simulink model "Model_1_PI_Gain_Test"  (R2017b)
settings: Solver=VariableStepAuto  StartTime=0.0  StopTime=1  MaxStep=1e-5  RelTol=1e-3  EnableMultiTasking=on
values from neighbouring files (symbols this model uses):
  Gain_I = 1    [Model_1_init.m]    (also in Model_2_init.m = 26.84; Model_3_init.m = 26.84)
  Gain_P = 1    [Model_1_init.m]    (also in Model_2_init.m = 7.74; Model_3_init.m = 7.74)
  Id_reference = -50    [Model_1_init.m]
  Iq_reference = 100    [Model_1_init.m]
  Lambda_m = 0.2205    [Model_1_init.m]    (also in Model_2_init.m; Model_3_init.m)
  Ld = 1.7e-3    (= 0.0017)    [Model_1_init.m]    (also in Model_2_init.m; Model_3_init.m)
  Lq = 3.2e-3    (= 0.0032)    [Model_1_init.m]    (also in Model_2_init.m; Model_3_init.m)
  Polepairs = 4    [Model_1_init.m]    (also in Model_2_init.m; Model_3_init.m)
  Rs = 0.02    [Model_1_init.m]    (also in Model_2_init.m; Model_3_init.m)
libraries: powerlib x19, simulink x5, powerlib_meascontrol x1
settings Model: SimulationMode=accelerator  Creator=dakaihu  LastModifiedBy=proso
settings DataIOCC: LimitDataPoints=on
settings OptimizationCC: LifeSpan=inf
settings DebuggingCC: AllowSymbolicDim=off  SFUnexpectedBacktrackingDiag=warning  SFNoUnconditionalDefaultTransitionDiag=warning  SFExecutionAtInitializationDiag=none
settings ModelReferenceCC: PropagateSignalLabelsOutOfModel=off
settings CodeAppCC: StateflowObjectComments=on
settings GRTTargetCC: TargetLangStandard=C89/C90 (ANSI)
settings ConfigComp: CovMetricSettings=dw  CovSaveCumulativeToWorkspaceVar=on  CovSaveSingleToWorkspaceVar=on  CovExternalEMLEnable=off
settings SimscapeCC: SimscapeNormalizeSystem=off

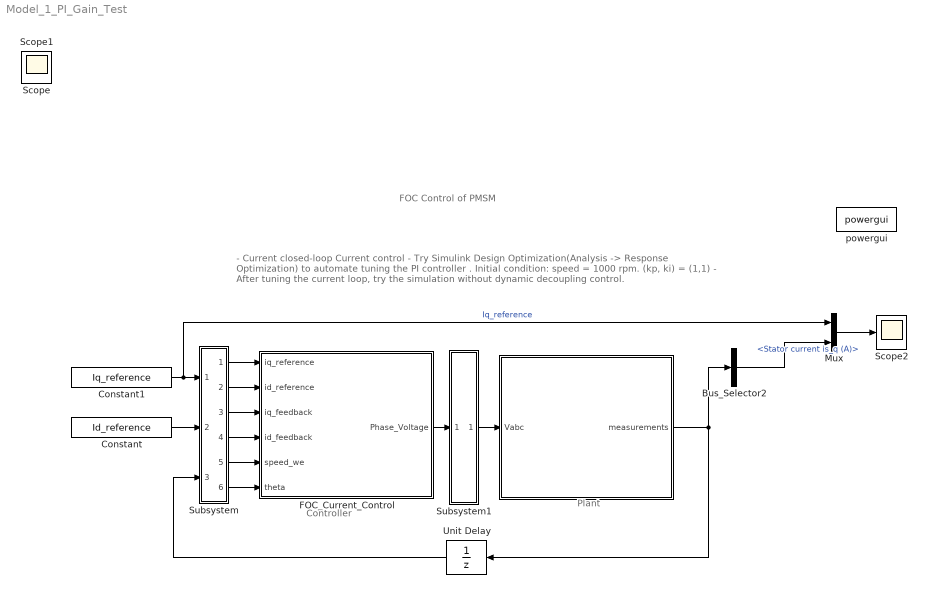
== system Model_1_PI_Gain_Test ==
  note: - Current closed-loop Current control
      | - Try Simulink Design Optimization(Analysis -> Response Optimization) to automate tuning the PI controller .  Initial condition: speed = 1000 rpm. (kp, ki) = (1,1)
      | - After tuning the current loop, try the simulation without dynamic decoupling control.
  note: Controller
  note: Plant
  note: FOC Control of PMSM
  " " : Subsystem
  Bus_Selector2 : BusSelector  OutputSignals=Stator current is_q (A)
  Constant : Constant  Value=Id_reference
  Constant1 : Constant  Value=Iq_reference  VectorParams1D=off
  FOC_Current_Control : Subsystem
  Mux : Mux  Inputs=2
  Scope2 : Scope
  Subsystem : Subsystem
      mask Display: fprintf('C/D')
  Subsystem1 : Subsystem
      mask Display: fprintf('D/C')
  Unit Delay : UnitDelay  SampleTime=1e-4
  powergui : powerlib/powergui  SimulationMode=Continuous  SampleTime=1e-5  frequency=60  Iterations=50  frequencyindice=0  Pbase=100e6  ErrMax=1e-4  UnitsV=kV  UnitsW=MW  buscounter=0  FunctionMessages=off  echomessages=off  EnableUseOfTLC=off  CurrentSourceSwitches=off  DisableSnubberDevices=off  DisableRonSwitches=off  DisableVfSwitches=off  DisplayEquations=off  SolverType=Tustin/Backward Euler (TBE)  Interpol=off  ExternalGateDelay=off  methode=off  Ts=100  x0status=blocks  SPID=on  SwTol=0  HookPort=off  RestoreLinks=warning  ResistiveCurrentMeasurement=off  Frange=[0:2:500]  Ylog=off  Xlog=on  ShowGrid=off  save=off  variable=ZData  structure=0  ZoomFFT=on  StartTime=0.0  cycles=1  DisplayStyle=1  fundamental=60  FreqAxis=off  MaxFrequency=1000  frequencyindicesteady=1  RmsSteady=1  display=off
  Scope : Scope
  Scope1 : Scope
  wires:
  FOC_Current_Control/1(Phase_Voltage) -> Subsystem1/1(In1)
  " "/1(measurements) -> Unit Delay/1, Bus_Selector2/1
  Subsystem/3(Out2) -> FOC_Current_Control/3(iq_feedback)
  Subsystem/4(Out3) -> FOC_Current_Control/4(id_feedback)
  Subsystem1/1(Out1) -> " "/1(Vabc)
  Unit Delay/1 -> Subsystem/3(PMSM_Measurements)
  Subsystem/5(Out1) -> FOC_Current_Control/5(speed_we)
  Subsystem/6(Out4) -> FOC_Current_Control/6(theta)
  Mux/1 -> Scope2/1
  Bus_Selector2/1 -> Mux/2  "<Stator current is_q (A)>"
  Constant/1 -> Subsystem/2(id_ref)
  Constant1/1 -> Mux/1, Subsystem/1(iq_ref)  "Iq_reference"
  Subsystem/1(Out6) -> FOC_Current_Control/1(iq_reference)
  Subsystem/2(Out5) -> FOC_Current_Control/2(id_reference)

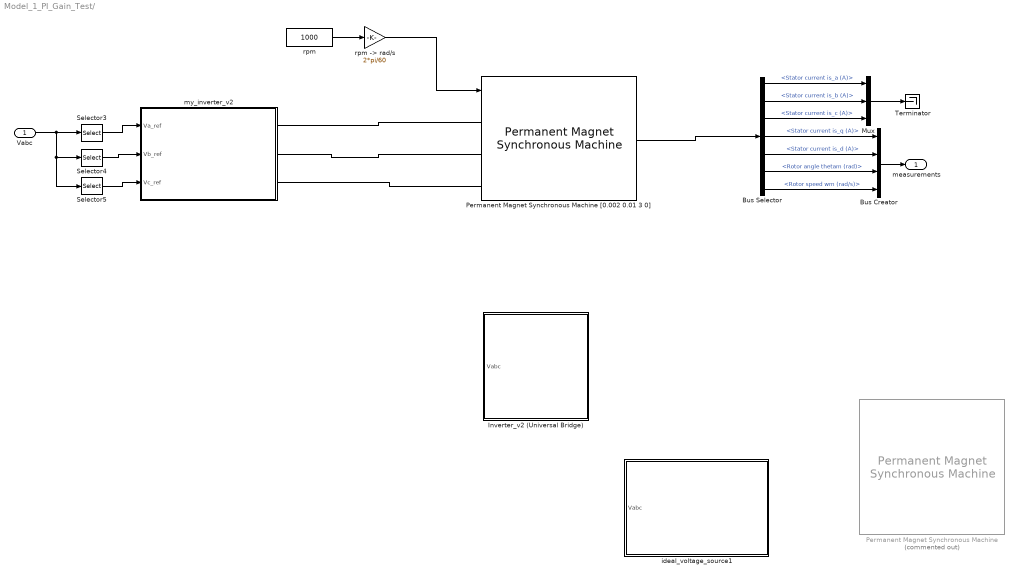
== system Model_1_PI_Gain_Test/  ==
  Vabc : Inport
  " Inverter_v2 (Universal Bridge)" : Subsystem
  Bus Creator : BusCreator  Inputs=4
  Bus Selector : BusSelector  OutputSignals=Stator current is_a (A),Stator current is_b (A),Stator current is_c (A),Stator current is_q (A),Stator current is_d (A),Rotor angle thetam (rad),Rotor speed wm (rad/s)
  Mux : Mux  Inputs=3
  Permanent Magnet Synchronous Machine : powerlib/Machines/Permanent Magnet Synchronous Machine  Commented=on  NbPhases=3  FluxDistribution=Sinusoidal  RotorType=Salient-pole  MechanicalLoad=Speed w  PresetModel=No  ShowDetailedParameters=on  MeasurementBus=off  Resistance=Rs  Inductance=8.5e-3  dqInductances=[Ld,Lq]  La=[Ld,Lq]  MachineConstant=Flux linkage established by magnets (V.s)  Flux=Lambda_m  VoltageCst=159.9771  TorqueCst=1.323  Flat=120  Mechanical=[0.0027 0.0004924 4 0]  PolePairs=Polepairs  InitialConditions=[0,0.01,3,0]  InitialConditions5ph=[0 0 0 0 0 0]  TsPowergui=0  TsBlock=-1  RefAngle=90 degrees behind phase A axis (modified Park)
      settings: SourceProductName=Simscape Power Systems
  Permanent Magnet Synchronous Machine [0.002 0.01 3 0] : powerlib/Machines/Permanent Magnet Synchronous Machine  NbPhases=3  FluxDistribution=Sinusoidal  RotorType=Salient-pole  MechanicalLoad=Speed w  PresetModel=No  ShowDetailedParameters=on  MeasurementBus=off  Resistance=Rs  Inductance=8.5e-3  dqInductances=[Ld,Lq]  La=0.000395  MachineConstant=Flux linkage established by magnets (V.s)  Flux=Lambda_m  VoltageCst=159.9771  TorqueCst=1.323  Flat=120  Mechanical=[0.0027 0.001 4 0]  PolePairs=Polepairs  InitialConditions=[0,0, 0,0]  InitialConditions5ph=[0 0 0 0 0 0]  TsPowergui=0  TsBlock=-1  RefAngle=Aligned with phase A axis (original Park)
  Selector3 : Selector  InputPortWidth=3  IndexOptions=Index vector (dialog)  Indices=[1]  OutputSizes=1
  Selector4 : Selector  InputPortWidth=3  IndexOptions=Index vector (dialog)  Indices=2  OutputSizes=1
  Selector5 : Selector  InputPortWidth=3  IndexOptions=Index vector (dialog)  Indices=3  OutputSizes=1
  Terminator : Terminator
  ideal_voltage_source1 : Subsystem  VariantControl=variantPwm == enumPwm.behavior
  my_inverter_v2 : Subsystem
  rpm : Constant  Value=1000
  "rpm -> rad/s" : Gain  Gain=2*pi/60
  measurements : Outport
  wires:
  rpm/1 -> "rpm -> rad/s"/1
  Bus Selector/4 -> Bus Creator/1  "<Stator current is_q (A)>"
  Bus Selector/5 -> Bus Creator/2  "<Stator current is_d (A)>"
  Bus Selector/6 -> Bus Creator/3  "<Rotor angle thetam (rad)>"
  Bus Creator/1 -> measurements/1
  Bus Selector/1 -> Mux/1  "<Stator current is_a (A)>"
  Bus Selector/2 -> Mux/2  "<Stator current is_b (A)>"
  Bus Selector/3 -> Mux/3  "<Stator current is_c (A)>"
  Mux/1 -> Terminator/1
  Permanent Magnet Synchronous Machine [0.002 0.01 3 0]/1 -> Bus Selector/1
  Bus Selector/7 -> Bus Creator/4  "<Rotor speed wm (rad/s)>"
  Vabc/1 -> Selector5/1, Selector4/1, Selector3/1
  Selector4/1 -> my_inverter_v2/2(Vb_ref)
  Selector3/1 -> my_inverter_v2/1(Va_ref)
  Selector5/1 -> my_inverter_v2/3(Vc_ref)
  "rpm -> rad/s"/1 -> Permanent Magnet Synchronous Machine [0.002 0.01 3 0]/1
  connections:
  my_inverter_v2/RConn1 -- Permanent Magnet Synchronous Machine [0.002 0.01 3 0]/LConn1
  my_inverter_v2/RConn2 -- Permanent Magnet Synchronous Machine [0.002 0.01 3 0]/LConn2
  my_inverter_v2/RConn3 -- Permanent Magnet Synchronous Machine [0.002 0.01 3 0]/LConn3

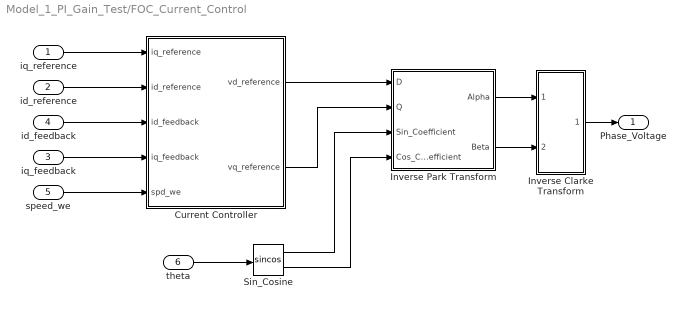
== system Model_1_PI_Gain_Test/FOC_Current_Control ==
  iq_reference : Inport  SampleTime=1e-4
  id_reference : Inport  Port=2  SampleTime=1e-4
  iq_feedback : Inport  Port=3  SampleTime=1e-4
  id_feedback : Inport  Port=4  SampleTime=1e-4
  speed_we : Inport  Port=5  SampleTime=1e-4
  theta : Inport  Port=6  SampleTime=1e-4
  Current Controller : Subsystem
  Inverse Clarke Transform : Subsystem
  Inverse Park Transform : Subsystem
  Sin_Cosine : Trigonometry  Operator=sincos
  Phase_Voltage : Outport  SampleTime=1e-4
  wires:
  Inverse Clarke Transform/1(ABC) -> Phase_Voltage/1
  Sin_Cosine/2 -> Inverse Park Transform/4(Cos_Coefficient)
  Sin_Cosine/1 -> Inverse Park Transform/3(Sin_Coefficient)
  theta/1 -> Sin_Cosine/1
  Current Controller/2(vq_reference) -> Inverse Park Transform/2(Q)
  Current Controller/1(vd_reference) -> Inverse Park Transform/1(D)
  Inverse Park Transform/1(Alpha) -> Inverse Clarke Transform/1(Alpha)
  Inverse Park Transform/2(Beta) -> Inverse Clarke Transform/2(Beta)
  id_feedback/1 -> Current Controller/3(id_feedback)
  iq_feedback/1 -> Current Controller/4(iq_feedback)
  speed_we/1 -> Current Controller/5(spd_we)
  iq_reference/1 -> Current Controller/1(iq_reference)
  id_reference/1 -> Current Controller/2(id_reference)

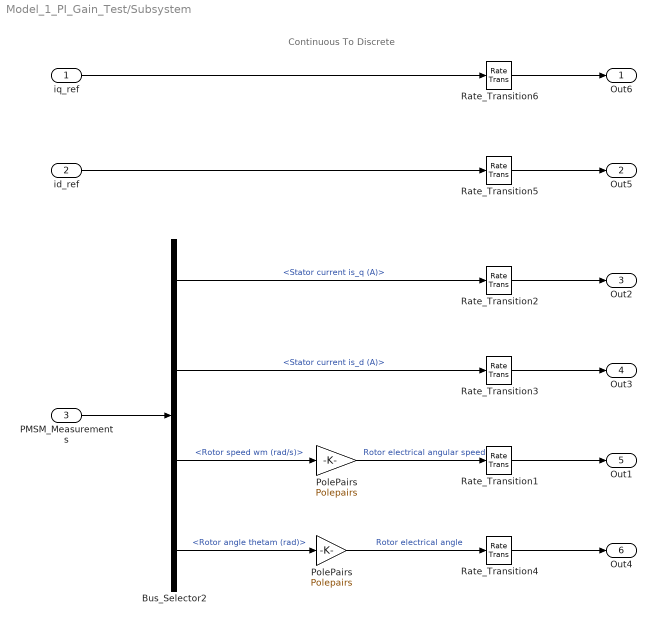
== system Model_1_PI_Gain_Test/Subsystem ==
  note: Continuous To Discrete
  iq_ref : Inport
  id_ref : Inport  Port=2
  PMSM_Measurements : Inport  Port=3
  Bus_Selector2 : BusSelector  OutputSignals=Stator current is_q (A),Stator current is_d (A),Rotor speed wm (rad/s),Rotor angle thetam (rad)
  PolePairs : Gain  Gain=Polepairs
  "PolePairs " : Gain  Gain=Polepairs
  Rate_Transition{1..6} (6 alike) : RateTransition  Integrity=off  Deterministic=off
  Out6 : Outport
  Out5 : Outport  Port=2
  Out2 : Outport  Port=3
  Out3 : Outport  Port=4
  Out1 : Outport  Port=5
  Out4 : Outport  Port=6
  wires:
  Rate_Transition4/1 -> Out4/1
  Bus_Selector2/2 -> Rate_Transition3/1  "<Stator current is_d (A)>"
  id_ref/1 -> Rate_Transition5/1
  iq_ref/1 -> Rate_Transition6/1
  Bus_Selector2/1 -> Rate_Transition2/1  "<Stator current is_q (A)>"
  Bus_Selector2/4 -> PolePairs/1  "<Rotor angle thetam (rad)>"
  PMSM_Measurements/1 -> Bus_Selector2/1
  PolePairs/1 -> Rate_Transition4/1  "Rotor electrical angle"
  Rate_Transition5/1 -> Out5/1
  Rate_Transition6/1 -> Out6/1
  Rate_Transition2/1 -> Out2/1
  Rate_Transition3/1 -> Out3/1
  Rate_Transition1/1 -> Out1/1
  Bus_Selector2/3 -> "PolePairs "/1  "<Rotor speed wm (rad/s)>"
  "PolePairs "/1 -> Rate_Transition1/1  "Rotor electrical angular speed"

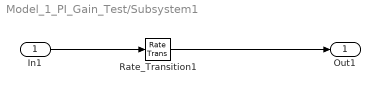
== system Model_1_PI_Gain_Test/Subsystem1 ==
  In1 : Inport
  Rate_Transition1 : RateTransition  Integrity=off
  Out1 : Outport
  wires:
  In1/1 -> Rate_Transition1/1
  Rate_Transition1/1 -> Out1/1

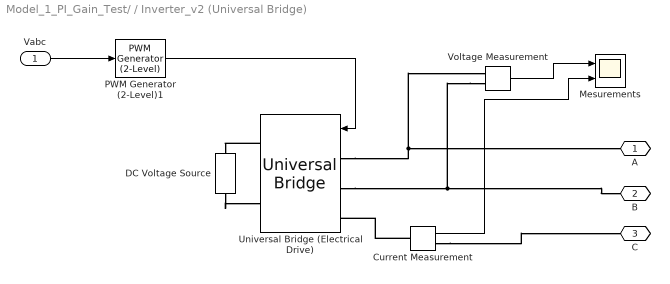
== system Model_1_PI_Gain_Test/ / Inverter_v2 (Universal Bridge) ==
  Vabc : Inport
  Current Measurement : powerlib/Measurements/Current Measurement  PhasorSimulation=off  OutputType=Complex  PSBequivalent=0
  DC Voltage Source : powerlib/Electrical Sources/DC Voltage Source  Amplitude=100  Measurements=None
  Mesurements : Scope  NumInputPorts=2
  PWM Generator (2-Level)1 : powerlib_meascontrol/Pulse & Signal Generators/PWM Generator (2-Level)  ModulatorType=Three-phase bridge (6 pulses)  ModulatorMode=Unsynchronized  Fc=27*60  Pc=90  nF=27  MinMax="[ -1  1 ]"  SamplingTechnique=Natural  ModulatingSignals=off  m=0.8  Freq=60  Phase=0  Ts=0  ShowCarrierOutport=off
      settings: SourceProductName=Simscape Power Systems
  Universal Bridge (Electrical Drive) : powerlib/Power Electronics/Universal Bridge  Arms=3  SnubberResistance=1e5  SnubberCapacitance=inf  Device=IGBT / Diodes  Ron=1e-3  Lon=0  ForwardVoltages="[  0  0  ]"  ForwardVoltage=0  GTOparameters=[ 10e-6 , 20e-6 ]  IGBTparameters=[ 1e-6 , 2e-6 ]  Measurements=None  Measurements_2=None  converterType=Rectifier
  Voltage Measurement : powerlib/Measurements/Voltage Measurement  PhasorSimulation=off  OutputType=Complex  PSBequivalent=0
  A : PMIOPort  Port=1  Side=Right
  B : PMIOPort  Port=2  Side=Right
  C : PMIOPort  Port=3  Side=Right
  wires:
  PWM Generator (2-Level)1/1 -> Universal Bridge (Electrical Drive)/1
  Vabc/1 -> PWM Generator (2-Level)1/1
  Voltage Measurement/1 -> Mesurements/1
  Current Measurement/1 -> Mesurements/2
  connections:
  Universal Bridge (Electrical Drive)/RConn1 -- DC Voltage Source/RConn1
  DC Voltage Source/LConn1 -- Universal Bridge (Electrical Drive)/RConn2
  Current Measurement/LConn1 -- Universal Bridge (Electrical Drive)/LConn3
  Universal Bridge (Electrical Drive)/LConn1 -- Voltage Measurement/LConn1 -- A/RConn1
  Voltage Measurement/LConn2 -- Universal Bridge (Electrical Drive)/LConn2 -- B/RConn1
  Current Measurement/RConn1 -- C/RConn1

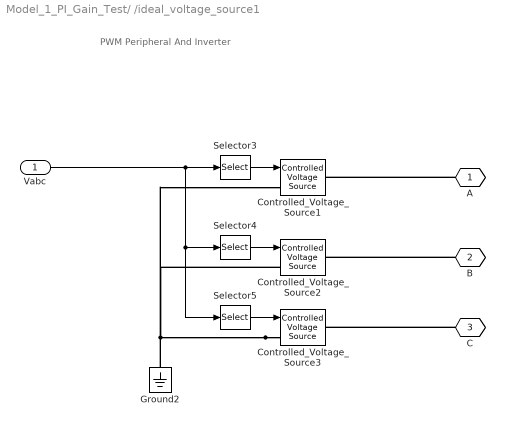
== system Model_1_PI_Gain_Test/ /ideal_voltage_source1 ==
  note: PWM Peripheral And Inverter
  Vabc : Inport
  Controlled_Voltage_Source1 : powerlib/Electrical Sources/Controlled Voltage Source  Initialize=off  Source_Type=DC  Amplitude=12  Phase=0  Frequency=0  Measurements=None
  Controlled_Voltage_Source2 : powerlib/Electrical Sources/Controlled Voltage Source  Initialize=off  Source_Type=DC  Amplitude=12  Phase=0  Frequency=0  Measurements=None
  Controlled_Voltage_Source3 : powerlib/Electrical Sources/Controlled Voltage Source  Initialize=off  Source_Type=DC  Amplitude=12  Phase=0  Frequency=0  Measurements=None
  Ground2 : powerlib/Elements/Ground  LConnTagsString=a
  Selector3 : Selector  InputPortWidth=3  IndexOptions=Index vector (dialog)  Indices=[1]  OutputSizes=1
  Selector4 : Selector  InputPortWidth=3  IndexOptions=Index vector (dialog)  Indices=2  OutputSizes=1
  Selector5 : Selector  InputPortWidth=3  IndexOptions=Index vector (dialog)  Indices=3  OutputSizes=1
  A : PMIOPort  Tag=PMCPort  Port=1  Side=Right
  B : PMIOPort  Tag=PMCPort  Port=2  Side=Right
  C : PMIOPort  Tag=PMCPort  Port=3  Side=Right
  wires:
  Vabc/1 -> Selector4/1, Selector5/1, Selector3/1
  Selector5/1 -> Controlled_Voltage_Source3/1
  Selector4/1 -> Controlled_Voltage_Source2/1
  Selector3/1 -> Controlled_Voltage_Source1/1
  connections:
  C/RConn1 -- Controlled_Voltage_Source3/RConn1
  B/RConn1 -- Controlled_Voltage_Source2/RConn1
  A/RConn1 -- Controlled_Voltage_Source1/RConn1
  Controlled_Voltage_Source3/LConn1 -- Controlled_Voltage_Source1/LConn1 -- Controlled_Voltage_Source2/LConn1 -- Ground2/LConn1

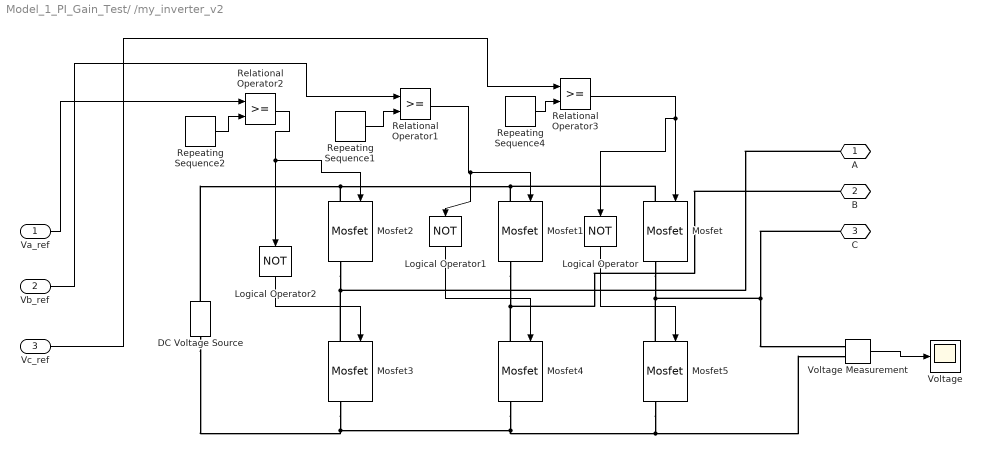
== system Model_1_PI_Gain_Test/ /my_inverter_v2 ==
  Va_ref : Inport
  Vb_ref : Inport  Port=2
  Vc_ref : Inport  Port=3
  DC Voltage Source : powerlib/Electrical Sources/DC Voltage Source  Amplitude=320  Measurements=None
  Logical Operator : Logic  Operator=NOT  AllPortsSameDT=off  OutDataTypeStr=boolean
  Logical Operator1 : Logic  Operator=NOT  AllPortsSameDT=off  OutDataTypeStr=boolean
  Logical Operator2 : Logic  Operator=NOT  AllPortsSameDT=off  OutDataTypeStr=boolean
  Mosfet{,1..5} (6 alike) : powerlib/Power Electronics/Mosfet  Ron=0.1  Lon=0  Rd=0.01  Vfd=0  IC=0  Rs=1e5  Cs=inf  Measurements=on
  Relational Operator1 : RelationalOperator  OutDataTypeStr=boolean  RndMeth=Simplest
  Relational Operator2 : RelationalOperator  OutDataTypeStr=boolean  RndMeth=Simplest
  Relational Operator3 : RelationalOperator  OutDataTypeStr=boolean  RndMeth=Simplest
  Repeating Sequence1 : simulink/Sources/Repeating Sequence  rep_seq_t="[0 (1/5000)/4  (1/5000)/2 (3/5000)/4 1/5000]"  rep_seq_y=[0 1 0 -1 0]
  Repeating Sequence2 : simulink/Sources/Repeating Sequence  rep_seq_t="[0 (1/5000)/4  (1/5000)/2 (3/5000)/4 1/5000]"  rep_seq_y=[0 1 0 -1 0]
  Repeating Sequence4 : simulink/Sources/Repeating Sequence  rep_seq_t="[0 (1/5000)/4  (1/5000)/2 (3/5000)/4 1/5000]"  rep_seq_y=[0 1 0 -1 0]
  Voltage : Scope
  Voltage Measurement : powerlib/Measurements/Voltage Measurement  PhasorSimulation=off  OutputType=Complex  PSBequivalent=0
  A : PMIOPort  Port=1  Side=Right
  B : PMIOPort  Port=2  Side=Right
  C : PMIOPort  Port=3  Side=Right
  wires:
  Relational Operator1/1 -> Mosfet1/1, Logical Operator1/1
  Vc_ref/1 -> Relational Operator3/1
  Logical Operator2/1 -> Mosfet3/1
  Va_ref/1 -> Relational Operator2/1
  Repeating Sequence4/1 -> Relational Operator3/2
  Repeating Sequence2/1 -> Relational Operator2/2
  Repeating Sequence1/1 -> Relational Operator1/2
  Relational Operator3/1 -> Mosfet/1, Logical Operator/1
  Relational Operator2/1 -> Mosfet2/1, Logical Operator2/1
  Vb_ref/1 -> Relational Operator1/1
  Logical Operator/1 -> Mosfet5/1
  Logical Operator1/1 -> Mosfet4/1
  Voltage Measurement/1 -> Voltage/1
  connections:
  Mosfet2/LConn1 -- Mosfet1/LConn1 -- Mosfet/LConn1 -- DC Voltage Source/RConn1
  Mosfet5/LConn1 -- Mosfet/RConn1 -- C/RConn1 -- Voltage Measurement/LConn1
  Mosfet3/LConn1 -- Mosfet2/RConn1 -- A/RConn1
  Mosfet5/RConn1 -- DC Voltage Source/LConn1 -- Mosfet3/RConn1 -- Mosfet4/RConn1 -- Voltage Measurement/LConn2
  Mosfet4/LConn1 -- Mosfet1/RConn1 -- B/RConn1

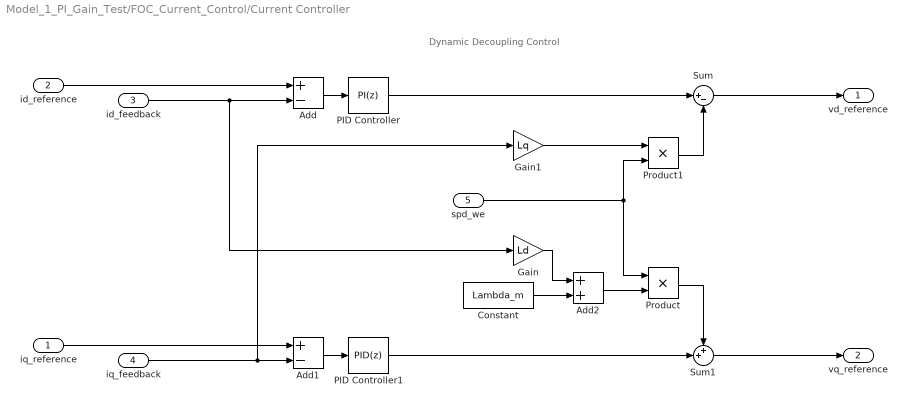
== system Model_1_PI_Gain_Test/FOC_Current_Control/Current Controller ==
  note: Dynamic Decoupling Control
  iq_reference : Inport  SampleTime=1e-4
  id_reference : Inport  Port=2  SampleTime=1e-4
  id_feedback : Inport  Port=3  SampleTime=1e-4
  iq_feedback : Inport  Port=4  SampleTime=1e-4
  spd_we : Inport  Port=5  SampleTime=1e-4
  Add : Sum  Inputs=+-
  Add1 : Sum  Inputs=+-
  Add2 : Sum
  Constant : Constant  Value=Lambda_m  SampleTime=1e-4
  Gain : Gain  Gain=Ld
  Gain1 : Gain  Gain=Lq
  PID Controller : simulink/Continuous/PID Controller  Controller=PI  TimeDomain=Discrete-time  SampleTime=-1  IntegratorMethod=Forward Euler  FilterMethod=Forward Euler  Form=Parallel  UseFilter=on  ControllerParametersSource=internal  P=Gain_P  I=Gain_I  D=0  N=100  InitialConditionSource=internal  InitialConditionForIntegrator=0  InitialConditionForFilter=0  ExternalReset=none  LimitOutput=off  UpperSaturationLimit=inf  LowerSaturationLimit=-inf  LinearizeAsGain=on  AntiWindupMode=none  Kb=1  TrackingMode=off  Kt=1  PParamMin=[]  PParamMax=[]  IParamMin=[]  IParamMax=[]  DParamMin=[]  DParamMax=[]  NParamMin=[]  NParamMax=[]  KbParamMin=[]  KbParamMax=[]  KtParamMin=[]  KtParamMax=[]  POutMin=[]  POutMax=[]  IOutMin=[]  IOutMax=[]  DOutMin=[]  DOutMax=[]  NOutMin=[]  NOutMax=[]  KbOutMin=[]  KbOutMax=[]  KtOutMin=[]  KtOutMax=[]  IntegratorOutMin=[]  IntegratorOutMax=[]  FilterOutMin=[]  FilterOutMax=[]  SumOutMin=[]  SumOutMax=[]  SumI1OutMin=[]  SumI1OutMax=[]  SumI2OutMin=[]  SumI2OutMax=[]  SumI3OutMin=[]  SumI3OutMax=[]  SumDOutMin=[]  SumDOutMax=[]  SaturationOutMin=[]  SaturationOutMax=[]  IntegratorContinuousStateAttributes=''  IntegratorStateMustResolveToSignalObject=off  IntegratorRTWStateStorageClass=Auto  FilterContinuousStateAttributes=''  FilterStateMustResolveToSignalObject=off  FilterRTWStateStorageClass=Auto  DifferentiatorICPrevScaledInput=0  DifferentiatorOutMin=[]  DifferentiatorOutMax=[]  InitialConditionSetting=State (most efficient)  FilterDiffOutCoefMin=[]  FilterDiffOutCoefMax=[]  SumDenOutMin=[]  SumDenOutMax=[]  SumNumOutMin=[]  SumNumOutMax=[]  ReciprocalOutMin=[]  ReciprocalOutMax=[]  DivideOutMin=[]  DivideOutMax=[]  TunerSelectOption=Transfer Function Based (PID Tuner App)
  PID Controller1 : simulink/Continuous/PID Controller  Controller=PID  TimeDomain=Discrete-time  SampleTime=-1  IntegratorMethod=Forward Euler  FilterMethod=Forward Euler  Form=Parallel  UseFilter=on  ControllerParametersSource=internal  P=Gain_P  I=Gain_I  D=0  N=100  InitialConditionSource=internal  InitialConditionForIntegrator=0  InitialConditionForFilter=0  ExternalReset=none  LimitOutput=off  UpperSaturationLimit=inf  LowerSaturationLimit=-inf  LinearizeAsGain=on  AntiWindupMode=none  Kb=1  TrackingMode=off  Kt=1  PParamMin=[]  PParamMax=[]  IParamMin=[]  IParamMax=[]  DParamMin=[]  DParamMax=[]  NParamMin=[]  NParamMax=[]  KbParamMin=[]  KbParamMax=[]  KtParamMin=[]  KtParamMax=[]  POutMin=[]  POutMax=[]  IOutMin=[]  IOutMax=[]  DOutMin=[]  DOutMax=[]  NOutMin=[]  NOutMax=[]  KbOutMin=[]  KbOutMax=[]  KtOutMin=[]  KtOutMax=[]  IntegratorOutMin=[]  IntegratorOutMax=[]  FilterOutMin=[]  FilterOutMax=[]  SumOutMin=[]  SumOutMax=[]  SumI1OutMin=[]  SumI1OutMax=[]  SumI2OutMin=[]  SumI2OutMax=[]  SumI3OutMin=[]  SumI3OutMax=[]  SumDOutMin=[]  SumDOutMax=[]  SaturationOutMin=[]  SaturationOutMax=[]  IntegratorContinuousStateAttributes=''  IntegratorStateMustResolveToSignalObject=off  IntegratorRTWStateStorageClass=Auto  FilterContinuousStateAttributes=''  FilterStateMustResolveToSignalObject=off  FilterRTWStateStorageClass=Auto  DifferentiatorICPrevScaledInput=0  DifferentiatorOutMin=[]  DifferentiatorOutMax=[]  InitialConditionSetting=State (most efficient)  FilterDiffOutCoefMin=[]  FilterDiffOutCoefMax=[]  SumDenOutMin=[]  SumDenOutMax=[]  SumNumOutMin=[]  SumNumOutMax=[]  ReciprocalOutMin=[]  ReciprocalOutMax=[]  DivideOutMin=[]  DivideOutMax=[]  TunerSelectOption=Transfer Function Based (PID Tuner App)
  Product : Product
  Product1 : Product
  Sum : Sum  Inputs=|+-
  Sum1 : Sum  Inputs=++|
  vd_reference : Outport  SampleTime=1e-4
  vq_reference : Outport  Port=2  SampleTime=1e-4
  wires:
  Sum/1 -> vd_reference/1
  PID Controller/1 -> Sum/1
  id_feedback/1 -> Gain/1, Add/2
  Add/1 -> PID Controller/1
  iq_feedback/1 -> Gain1/1, Add1/2
  id_reference/1 -> Add/1
  Add1/1 -> PID Controller1/1
  iq_reference/1 -> Add1/1
  Sum1/1 -> vq_reference/1
  PID Controller1/1 -> Sum1/2
  Gain/1 -> Add2/1
  Constant/1 -> Add2/2
  Add2/1 -> Product/2
  spd_we/1 -> Product1/2, Product/1
  Gain1/1 -> Product1/1
  Product1/1 -> Sum/2
  Product/1 -> Sum1/1

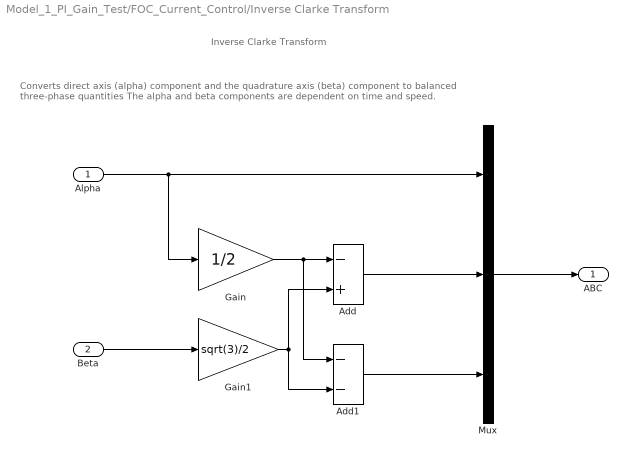
== system Model_1_PI_Gain_Test/FOC_Current_Control/Inverse Clarke Transform ==
  note: Inverse Clarke Transform
  note: Converts direct axis (alpha) component and the quadrature axis (beta) component to balanced three-phase quantities
      | The alpha and beta components are dependent on time and speed.
  Alpha : Inport
  Beta : Inport  Port=2
  Add : Sum  Inputs=-+  OutDataTypeStr=Inherit: Same as first input
  Add1 : Sum  Inputs=--  OutDataTypeStr=Inherit: Same as first input
  Gain : Gain  Gain=1/2
  Gain1 : Gain  Gain=sqrt(3)/2
  Mux : Mux  Inputs=3
  ABC : Outport
  wires:
  Beta/1 -> Gain1/1
  Mux/1 -> ABC/1
  Alpha/1 -> Mux/1, Gain/1
  Add1/1 -> Mux/3
  Gain1/1 -> Add1/2, Add/2
  Gain/1 -> Add1/1, Add/1
  Add/1 -> Mux/2

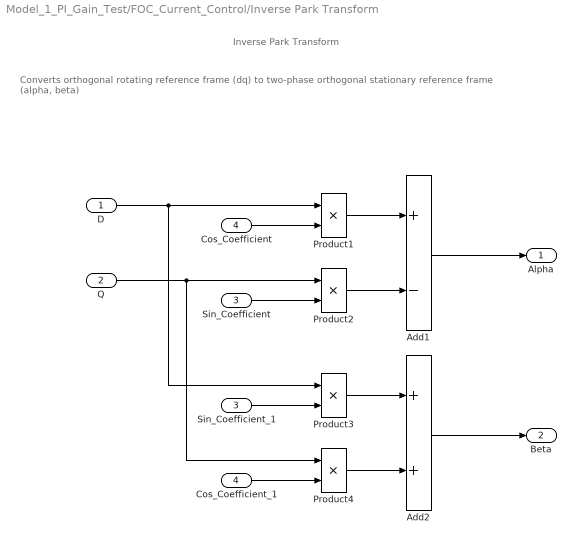
== system Model_1_PI_Gain_Test/FOC_Current_Control/Inverse Park Transform ==
  note: Converts orthogonal rotating reference frame (dq) to two-phase orthogonal stationary reference frame (alpha, beta)
  note: Inverse Park Transform
  D : Inport
  Q : Inport  Port=2
  Sin_Coefficient : Inport  Port=3
  Cos_Coefficient : Inport  Port=4
  Add1 : Sum  Inputs=+-  OutDataTypeStr=Inherit: Same as first input
  Add2 : Sum  OutDataTypeStr=Inherit: Same as first input
  Cos_Coefficient_1 : InportShadow  Port=4
  Product{1..4} (4 alike) : Product  RndMeth=Simplest
  Sin_Coefficient_1 : InportShadow  Port=3
  Alpha : Outport
  Beta : Outport  Port=2
  wires:
  Sin_Coefficient_1/1 -> Product3/2
  Product2/1 -> Add1/2
  Cos_Coefficient_1/1 -> Product4/2
  Add2/1 -> Beta/1
  Product3/1 -> Add2/1
  Add1/1 -> Alpha/1
  Product1/1 -> Add1/1
  Product4/1 -> Add2/2
  Sin_Coefficient/1 -> Product2/2
  D/1 -> Product3/1, Product1/1
  Q/1 -> Product2/1, Product4/1
  Cos_Coefficient/1 -> Product1/2
